simulink model "dsp_proj"  (R2015a)
settings: Solver=ode45  StartTime=0.0  StopTime=10.0  RelTol=1e-3
libraries: visionsources x1, visionsinks x1
settings Model: Creator=Jithendra HS  LastModifiedBy=Jithendra HS

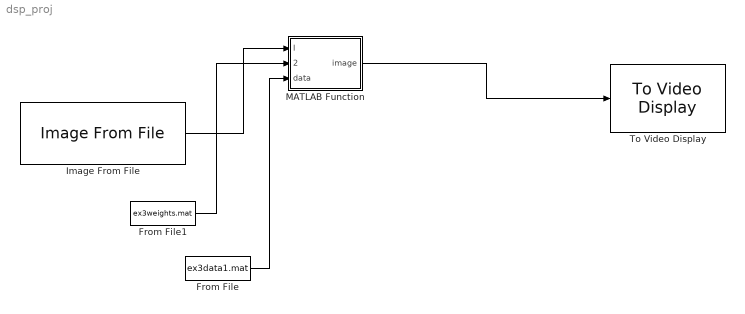
== system dsp_proj ==
  From File : FromFile  FileName=ex3data1.mat  SampleTime=0
  From File1 : FromFile  FileName=ex3weights.mat  SampleTime=0
  Image From File : visionsources/Image From File  Tag=vipblks_nd  FileName=C:\Users\Jithendra HS\Desktop\one1.jpg  imagePorts=One multidimensional signal  Ts=inf  ImageDataType=Inherit from input image  Signed=on  WordLength=16  sdImageDataType=uint(8)  FractionLengthMode=User-defined  FractionLength=15  OutPortLabels=R|G|B
  MATLAB Function : MATLAB Function  TreatAsAtomicUnit=on
  To Video Display : visionsinks/To Video Display  windowSizeMode=Normal  openAtMdlStart=on  fullScreen=off  videoWindowX=536805376  videoWindowY=536805376  saveWindowSize=off  videoWindowWidth=2147483647  videoWindowHeight=2147483647  inputColorFormat=RGB  inputType=Obsolete  imagePorts=One multidimensional signal  OutputDevice=On-screen video monitor  dataOrg=Column-major  isWindowOpen=off
  wires:
  From File1/1 -> MATLAB Function/2(weights)
  From File/1 -> MATLAB Function/3(data)
  Image From File/1 -> MATLAB Function/1(I)
  MATLAB Function/1(image) -> To Video Display/1

== matlab function dsp_proj/MATLAB Function ==
  data: I input; image output; weights input; data input
function image  = fcn(I,weights,data)


%% Setup the parameters you will use for this exercise
input_layer_size  = 400;  % 20x20 Input Images of Digits
hidden_layer_size = 25;   % 25 hidden units
num_labels = 10;          % 10 labels, from 1 to 10   
                          % (note that we have mapped "0" to label 10)

%% =========== Part 1: Loading and Visualizing Data =============
%  We start the exercise by first loading and visualizing the dataset. 
%  You will be working with a dataset that contains handwritten digits.
%

% Load Training Data
fprintf('Loading and Visualizing Data ...\n')

 %load('ex3data1.mat');
X=0;
s = size(X, 1);

% Randomly select 100 data points to display
sel=0;
sel = randperm(size(X, 1));
sel = sel(1:100);

image=(sel);

fprintf('Program paused. Press enter to continue.\n');
pause;

%% ================ Part 2: Loading Pameters ================
% In this part of the exercise, we load some pre-initialized 
% neural network parameters.

fprintf('\nLoading Saved Neural Network Parameters ...\n')

% Load the weights into variables Theta1 and Theta2
m=load('ex3weights.mat');

%% ================= Part 3: Implement Predict =================
%  After training the neural network, we would like to use it to predict
%  the labels. You will now implement the "predict" function to use the
%  neural network to predict the labels of the training set. This lets
%  you compute the training set accuracy.

theta1 = m.Theta1;
theta2 = m.Theta2;

pred = mypredict(theta1, theta2, X);

fprintf('\nTraining Set Accuracy: %f\n', mean(double(pred == y)) * 100);

fprintf('Program paused. Press enter to continue.\n');
pause;

%  To give you an idea of the network's output, you can also run
%  through the examples one at the a time to see what it is predicting.

%  Randomly permute examples
rp = randperm(s);
I=0;
I =imread('one1.JPG'); 
%m,n] = size(I);
%grayimage=rgb2gray(I);
%[a,b]=size(grayimage);
%J = imresize(grayimage, [20 20]);
%[x,y] = size(J);
%I2 = im2double(J);
%I3=reshape(I2,[1,400]);
disp(I);
imshow(I);
displayData(I(1,:));
    pred = predict(Theta1, Theta2,I(1,:));
   fprintf('\nNeural Network Prediction: %d (digit %d)\n', pred, mod(pred, 10));
y = u;
